simulink model "lift"  (R2024b)
settings: Solver=VariableStepAuto  StartTime=0.0  StopTime=inf  RelTol=1e-3
settings Model: Creator=Kumaresh Raj  LastModifiedBy=Kumaresh Raj

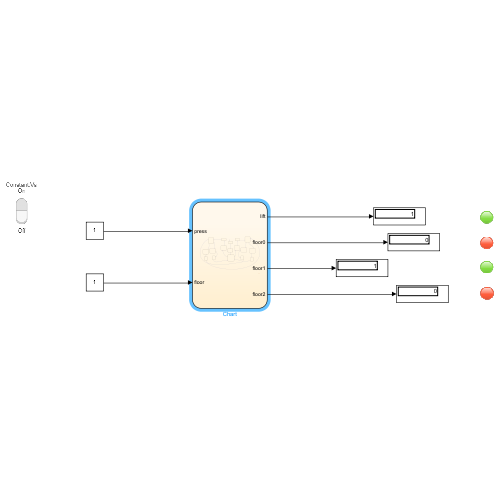
[thumbnail: Simulink's stored preview of the top-level diagram]
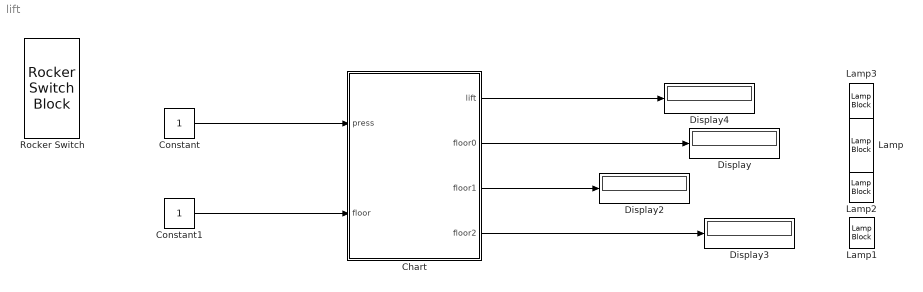
== system lift ==
  Chart : Stateflow chart  TreatAsAtomicUnit=on
  Constant : Constant
  Constant1 : Constant
  Display{,2..4} (4 alike) : Display
  Lamp{,1..3} (4 alike) : LampBlock  LabelPosition=Hide
  Rocker Switch : RockerSwitchBlock
      settings: Values={{'Off', 'On'}, [0 1]}
  wires:
  Constant/1 -> Chart/1(press)
  Constant1/1 -> Chart/2(floor)
  Chart/2(floor0) -> Display/1
  Chart/3(floor1) -> Display2/1
  Chart/4(floor2) -> Display3/1
  Chart/1(lift) -> Display4/1

== stateflow chart lift/Chart ==
  state second_floor
    entry:
    lift=1;
    floor2=1;
    during:
    floor0=0;
    floor1=0;
  state first_floor
    entry:
    lift=1;
    floor1=1;
    during:
    floor0=0;
    floor2=0;
  state close1
    lift=0;
  state close2
    lift=0;
  state close
    lift=0;
  state floor1
    entry:
    floor1=1;
    during:
    floor0=0;
  state floor2
    entry:
    floor2=1;
    during:
    floor0=0;
  state zerofloor
    entry:
    floor0=1;
    during:
    floor2=0;
  state firstfloor1
    entry:
    floor1=1;
    during:
    floor2=0;
  state zerofloor1
    entry:
    floor0=1;
    during:
    floor1=0;
  state open
    lift=1;
  state secondfloor1
    entry:
    floor2=1;
    during:
    floor1=0
  state groundfloor
    entry:
    floor0=1;
    during:
    floor1=0;
    floor2=0;
  state close3
    lift=0;
  state close4
    lift=0;
  state close6
    lift=0;
  state close5
    lift=0;
  close6 -> second_floor : after(15,sec)
  (default) -> close [order 1]
  close5 -> first_floor : after(15,sec)
  close1 -> first_floor : after(15,sec)
  close2 -> second_floor : after(15,sec)
  floor1 -> close1 : after(5,sec)
  floor2 -> close2 : after(5,sec)
  first_floor -> zerofloor1 : [floor==0]
  second_floor -> zerofloor [order 2] : [floor==0]
  second_floor -> firstfloor1 [order 1] : [floor==1]
  close -> open : [press==1]
  (default) -> secondfloor1 [order 2] : [floor==1]
  groundfloor -> floor1 [order 1] : [floor==1]
  groundfloor -> floor2 [order 2] : [floor==2]
  zerofloor -> close4 : after(5,sec)
  zerofloor1 -> close3 : after(5,sec)
  open -> groundfloor : [floor==0]
  firstfloor1 -> close5 : after(5,sec)
  secondfloor1 -> close6 : after(5,sec)
  close4 -> groundfloor : after(15,sec)
  close3 -> groundfloor : after(15,sec)
  data: lift output; press input; floor0 output; floor1 output; floor2 output; floor input
